simulink model "R7014E_Measure"  (R2025b)
settings: Solver=ode5  StartTime=0.0  StopTime=inf  RelTol=1e-3  EnableMultiTasking=on
undefined symbols (not defined in the file): Ad, Ao, At, Bd, Cd, g, h_0, h_1, h_1_V, h_2, h_2_V, National_Instruments, PCIe, Q, R, Ts
libraries: sldrtlib x2, simulink x2
settings Model: Creator=wolfgang  LastModifiedBy=Amar
settings Model: ModifiedHistory=|
  | Created an adjusted empty Simulink diagram for the lab assignments
  | in the course R0002E
settings SolverCC: AlgebraicLoopSolver=TrustRegion  AutoInsertRateTranBlk=on
settings DataIOCC: SaveFormat=Array  SignalLoggingSaveFormat=ModelDataLogs  SaveOutput=off  SignalLogging=off  DSMLogging=off  SaveTime=off  ReturnWorkspaceOutputs=off
settings OptimizationCC: ExpressionDepthLimit=2147483647.0  LifeSpan=inf
settings DebuggingCC: UnderspecifiedInitializationDetection=Classic  MergeDetectMultiDrivingBlocksExec=none  SolverPrmCheckMsg=warning  FcnCallInpInsideContextMsg=warning  UnconnectedInputMsg=warning  UnconnectedOutputMsg=warning  UnconnectedLineMsg=warning  StateNameClashWarn=warning  SFUnexpectedBacktrackingDiag=warning  SFNoUnconditionalDefaultTransitionDiag=warning  SFExecutionAtInitializationDiag=none  ArithmeticOperatorsInVariantConditions=warning
settings HardwareCC: ProdBitPerPointer=32.0  ProdBitPerSizeT=32.0  ProdBitPerPtrDiffT=32.0  ProdLargestAtomicFloat=None  ProdIntDivRoundTo=Undefined  ProdEndianess=Unspecified  ProdWordSize=32.0  ProdHWDeviceType=32-bit Generic
settings ModelReferenceCC: EnableRefExpFcnMdlSchedulingChecks=on  PropagateSignalLabelsOutOfModel=off
settings SFSimCC: SimUseLocalCustomCode=off  CustomCodeUndefinedFunction=UseInterfaceOnly
settings RTWCC: RTWUseLocalCustomCode=off  GPUComputeCapability=3.5
settings CodeAppCC: StateflowObjectComments=on
settings GRTTargetCC: TargetLangStandard=C89/C90 (ANSI)
settings ConfigComp: CovMetricSettings=dw  CovSaveCumulativeToWorkspaceVar=on  CovSaveSingleToWorkspaceVar=on  CovExternalEMLEnable=off  CovSFcnEnable=off

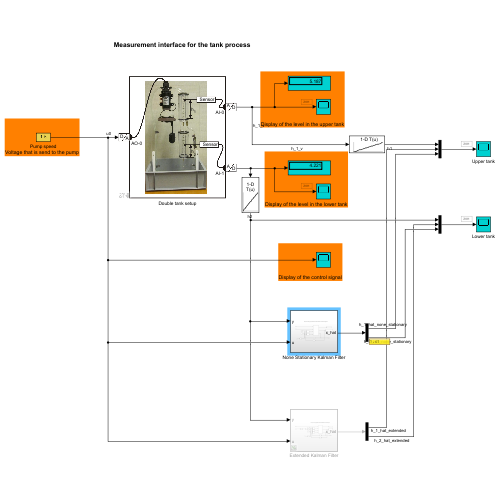
[thumbnail: Simulink's stored preview of the top-level diagram]
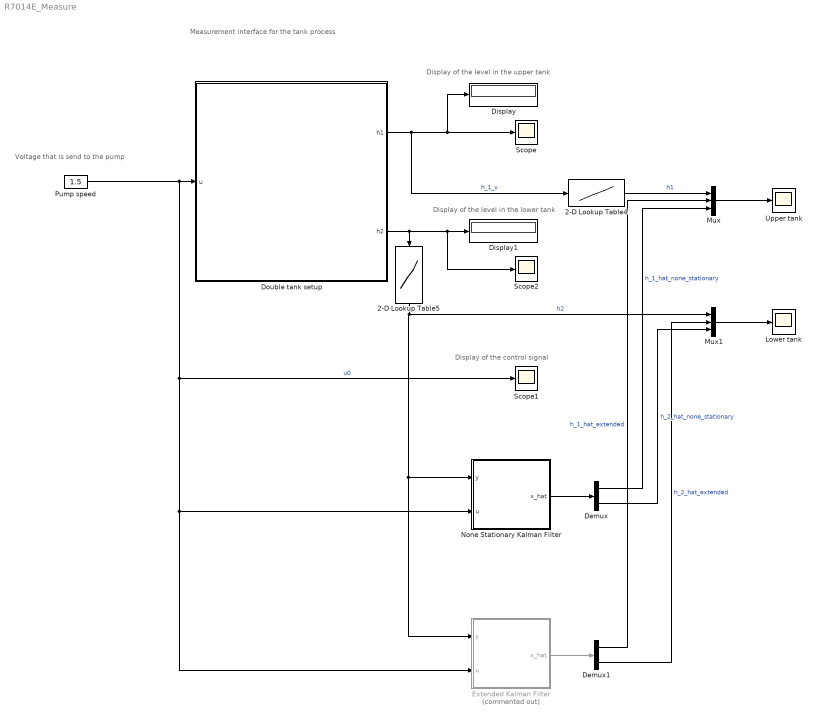
== system R7014E_Measure ==
  note: Measurement interface for the tank process
  note: Voltage that is send to the pump
  note: Display of the level in the upper tank
  note: Display of the control signal
  note: Display of the level in the lower tank
  2-D Lookup Table4 : Lookup_n-D  NumberOfTableDimensions=1  BreakpointsForDimension1=x  BreakpointsForDimension2=[1:3]  Table=y  RndMeth=Simplest  mask{x=h_1_V, y=h_1}
      mask prompts: x "Values on x-axis"; y "Values on y-axis"
  2-D Lookup Table5 : Lookup_n-D  NumberOfTableDimensions=1  BreakpointsForDimension1=x  BreakpointsForDimension2=[1:3]  Table=y  RndMeth=Simplest  mask{x=h_2_V, y=h_2}
      mask prompts: x "Values on x-axis"; y "Values on y-axis"
  Demux : Demux  Outputs=2
  Demux1 : Demux  Outputs=2
  Display : Display
  Display1 : Display
  Double tank setup : Subsystem  AncestorBlock=R0002E_lib/Double tank setup  mask(Realtime interface for the tank process){ts=Ts, h1_ch=0, h2_ch=1, u_ch=0}
      mask prompts: ts "Sample time"; h1_ch "A/D Channel for upper tank"; h2_ch "A/D Channel for lower tank"; u_ch "D/A Channel for pump"
      mask help:
      | This block represents the physical interface from the computer to the tank process.
      |
      | The input u is the voltage that is provided for the pump, the output h1 is the measured level in the upper tank in [V] and the output h2 is the
      | measured level in the lower tank in [V].
      |
      | You need to provide the sample rate at which the voltage to the pump is updated and the level measurements are sampled. The sample rate should not be less than 0.02 seconds.
      settings: LibrarySourceBlock=R0002E_lib/Double tank setup
      mask Display:
      | x=363;
      | y=381;
      | image(imread('tank_icon.jpg'));
      | text(250/x,309/y,'Sensor');
      | text(260/x,169/y,'Sensor');
      | text(335/x,289/y,'A');
      | text(351/x,283/y,'D');
      | text(335/x,100/y,'A');
      | text(351/x,95/y,'D');
      | text(22/x,187/y,'A');
      | text(5/x,195/y,'D');
      | text(225/x,278/y,'h_1','texmode','on');
      | text(225/x,146/y,'h_2','texmode','on');
      | text(300/x,270/y,sprintf('AI-%d',h1_ch));
      | text(300/x,80/y,sprintf('AI-%d',h2_ch));
      | text(40/x,173/y,sprintf('AO-%d',u_ch));
  Extended Kalman Filter : Subsystem  Commented=on
  Lower tank : Scope
      settings: SampleTime=0.1  TimeSpan=200  ActiveDisplayYMinimum=-4.8844046976277262  ActiveDisplayYMaximum=17.672626579116233  DataLoggingVariableName=ScopeData3  DataLoggingSaveFormat=Array
  Mux : Mux  Inputs=3
  Mux1 : Mux  Inputs=3
  None Stationary Kalman Filter : Subsystem
  Pump speed : Constant  Value=1.5
  Scope : Scope
      settings: SampleTime=0.1  TimeSpan=200  ActiveDisplayYMinimum=-1  ActiveDisplayYMaximum=1  DataLoggingSaveFormat=Array
  Scope1 : Scope
      settings: SampleTime=0.1  TimeSpan=200  ActiveDisplayYMinimum=0  DataLoggingSaveFormat=Array
  Scope2 : Scope
      settings: SampleTime=0.1  TimeSpan=200  ActiveDisplayYMinimum=0  ActiveDisplayYMaximum=20  DataLoggingVariableName=ScopeData2  DataLoggingSaveFormat=Array
  Upper tank : Scope
      settings: SampleTime=0.1  TimeSpan=200  ActiveDisplayYMinimum=-11.086400420135282  ActiveDisplayYMaximum=21.20768858424583  DataLoggingVariableName=ScopeData4  DataLoggingSaveFormat=Array
  wires:
  Pump speed/1 -> Extended Kalman Filter/2(u), None Stationary Kalman Filter/2(u), Scope1/1, Double tank setup/1(u)  "u0"
  Double tank setup/1(h1) -> 2-D Lookup Table4/1, Display/1, Scope/1  "h_1_v"
  Double tank setup/2(h2) -> 2-D Lookup Table5/1, Scope2/1, Display1/1
  None Stationary Kalman Filter/1(x_hat) -> Demux/1
  Demux/1 -> Mux/3  "h_1_hat_none_stationary"
  Demux/2 -> Mux1/3  "h_2_hat_none_stationary"
  Mux1/1 -> Lower tank/1
  Mux/1 -> Upper tank/1
  Extended Kalman Filter/1(x_hat) -> Demux1/1
  Demux1/1 -> Mux/2  "h_1_hat_extended"
  Demux1/2 -> Mux1/2  "h_2_hat_extended"
  2-D Lookup Table4/1 -> Mux/1  "h1"
  2-D Lookup Table5/1 -> Extended Kalman Filter/1(y), None Stationary Kalman Filter/1(y), Mux1/1  "h2"

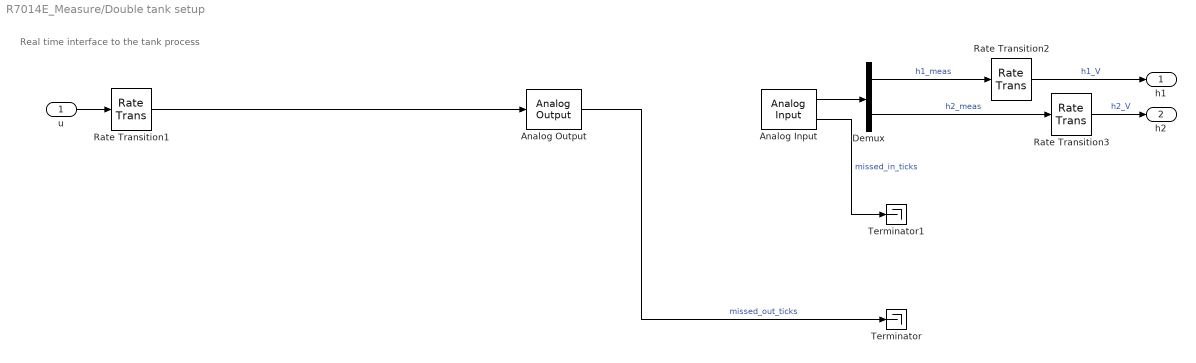
== system R7014E_Measure/Double tank setup ==
  note: Real time interface to the tank process
  u : Inport
  Analog Input : sldrtlib/Analog Input  SampleTime=ts  MaxMissedTicks=500000000  ShowMissedTicks=on  YieldWhenWaiting=off  DrvName=National_Instruments/PCIe-6321  DrvAddress=4294967295  DrvOptions=[0 0 0 0 0 0 0]  Channels=[h1_ch+1,h2_ch+1]  RangeMode=1  VoltRange=1  DataType=1
      settings: AttributesFormatString=National Instruments\nPCIe-6321 [auto]
  Analog Output : sldrtlib/Analog Output  SampleTime=ts  MaxMissedTicks=500000000  ShowMissedTicks=on  YieldWhenWaiting=off  DrvName=National_Instruments/PCIe-6321  DrvAddress=4294967295  DrvOptions=[0 0 0 0 0 0 0]  Channels=u_ch+1  RangeMode=1  VoltRange=1  InitialValue=0  FinalValue=0
      settings: AttributesFormatString=National Instruments\nPCIe-6321 [auto]
  Demux : Demux  Outputs=2
  Rate Transition1 : RateTransition  OutPortSampleTime=ts
  Rate Transition2 : RateTransition
  Rate Transition3 : RateTransition
  Terminator : Terminator
  Terminator1 : Terminator
  h1 : Outport
  h2 : Outport  Port=2
  wires:
  Rate Transition1/1 -> Analog Output/1
  Rate Transition3/1 -> h2/1  "h2_V"
  Rate Transition2/1 -> h1/1  "h1_V"
  Analog Input/2 -> Terminator1/1  "missed_in_ticks"
  Demux/2 -> Rate Transition3/1  "h2_meas"
  Demux/1 -> Rate Transition2/1  "h1_meas"
  Analog Input/1 -> Demux/1
  Analog Output/1 -> Terminator/1  "missed_out_ticks"
  u/1 -> Rate Transition1/1

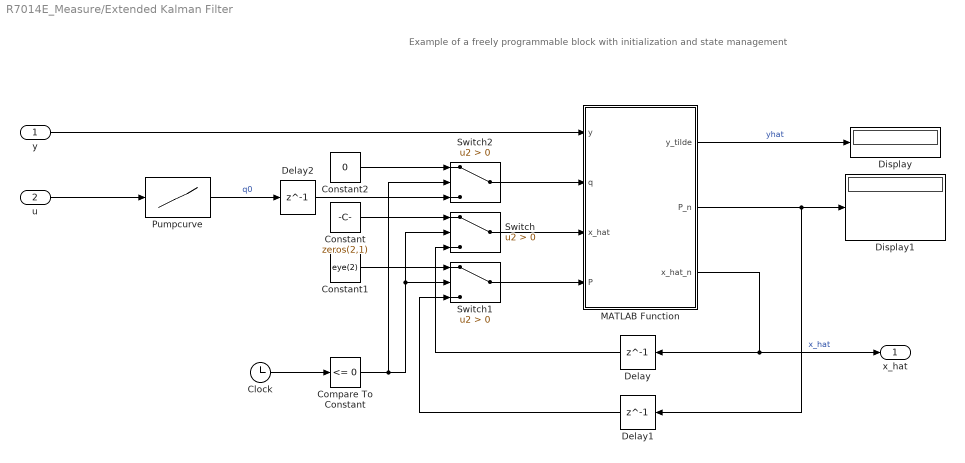
== system R7014E_Measure/Extended Kalman Filter ==
  note: Example of a freely programmable block with initialization and state management
  y : Inport
  u : Inport  Port=2
  Clock : Clock
  Compare To Constant : simulink/Logic and Bit Operations/Compare To Constant  relop=<=  const=0  OutDataTypeStr=boolean
  Constant : Constant  Value=zeros(2,1)
  Constant1 : Constant  Value=eye(2)
  Constant2 : Constant  Value=0
  Delay : Delay  DelayLength=1  InitialCondition=0
  Delay1 : Delay  DelayLength=1  InitialCondition=0
  Delay2 : Delay  DelayLength=1  InitialCondition=0
  Display : Display
  Display1 : Display
  MATLAB Function : MATLAB Function  TreatAsAtomicUnit=on
  Pumpcurve : Lookup_n-D  NumberOfTableDimensions=1  BreakpointsForDimension1=x  BreakpointsForDimension2=[1:3]  Table=y  RndMeth=Simplest  mask{x=[0.5,1,1.5,2,2.5,3,3.5,5,8,10], y=[16.47,20.75,24.52,27.63,30.06,32.49,34.80,40.28,48.24,52.43]}
      mask prompts: x "Values on x-axis"; y "Values on y-axis"
  Switch : Switch  Criteria=u2 > Threshold  SaturateOnIntegerOverflow=off  InputSameDT=off
  Switch1 : Switch  Criteria=u2 > Threshold  SaturateOnIntegerOverflow=off  InputSameDT=off
  Switch2 : Switch  Criteria=u2 > Threshold  SaturateOnIntegerOverflow=off  InputSameDT=off
  x_hat : Outport  PortDimensions=2
  wires:
  Delay/1 -> Switch/3
  Switch/1 -> MATLAB Function/3(x_hat)
  Constant1/1 -> Switch1/1
  Compare To Constant/1 -> Switch2/2, Switch/2, Switch1/2
  Constant/1 -> Switch/1
  MATLAB Function/1(y_tilde) -> Display/1  "yhat"
  MATLAB Function/2(P_n) -> Delay1/1, Display1/1
  Clock/1 -> Compare To Constant/1
  Switch1/1 -> MATLAB Function/4(P)
  y/1 -> MATLAB Function/1(y)
  Delay1/1 -> Switch1/3
  Switch2/1 -> MATLAB Function/2(q)
  Constant2/1 -> Switch2/1
  Delay2/1 -> Switch2/3
  Pumpcurve/1 -> Delay2/1  "q0"
  u/1 -> Pumpcurve/1
  MATLAB Function/3(x_hat_n) -> Delay/1, x_hat/1  "x_hat"

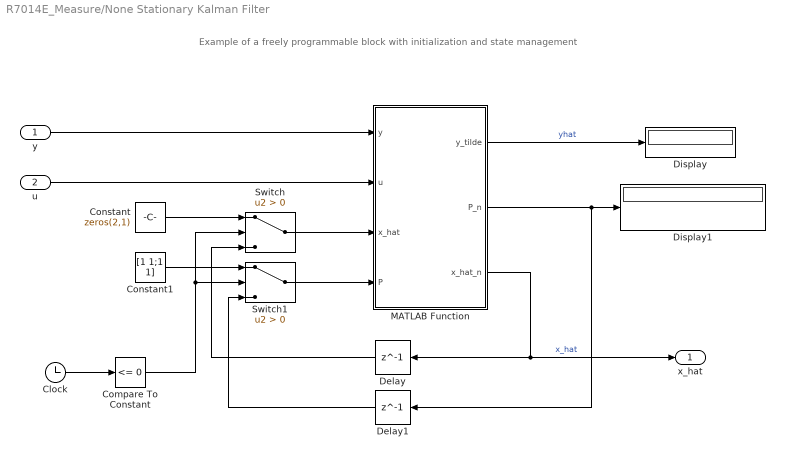
== system R7014E_Measure/None Stationary Kalman Filter ==
  note: Example of a freely programmable block with initialization and state management
  y : Inport
  u : Inport  Port=2
  Clock : Clock
  Compare To Constant : simulink/Logic and Bit Operations/Compare To Constant  relop=<=  const=0  OutDataTypeStr=boolean
  Constant : Constant  Value=zeros(2,1)
  Constant1 : Constant  Value=[1 1;1 1]
  Delay : Delay  DelayLength=1  InitialCondition=0
  Delay1 : Delay  DelayLength=1  InitialCondition=0
  Display : Display
  Display1 : Display
  MATLAB Function : MATLAB Function  TreatAsAtomicUnit=on
  Switch : Switch  Criteria=u2 > Threshold  SaturateOnIntegerOverflow=off  InputSameDT=off
  Switch1 : Switch  Criteria=u2 > Threshold  SaturateOnIntegerOverflow=off  InputSameDT=off
  x_hat : Outport  PortDimensions=2
  wires:
  Delay/1 -> Switch/3
  Switch/1 -> MATLAB Function/3(x_hat)
  Constant1/1 -> Switch1/1
  Compare To Constant/1 -> Switch1/2, Switch/2
  MATLAB Function/3(x_hat_n) -> x_hat/1, Delay/1  "x_hat"
  Constant/1 -> Switch/1
  MATLAB Function/1(y_tilde) -> Display/1  "yhat"
  MATLAB Function/2(P_n) -> Display1/1, Delay1/1
  Clock/1 -> Compare To Constant/1
  Switch1/1 -> MATLAB Function/4(P)
  y/1 -> MATLAB Function/1(y)
  Delay1/1 -> Switch1/3
  u/1 -> MATLAB Function/2(u)

== matlab function R7014E_Measure/None Stationary Kalman Filter/MATLAB Function ==
  data: y input; u input; x_hat input; y_tilde output; P input; P_n output; x_hat_n output; Ad parameter; Bd parameter; Cd parameter; Q parameter; R parameter
function [y_tilde, P_n, x_hat_n] = fcn(y, u, x_hat, P, Ad, Bd, Cd, Q, R)

% Predict
x_hat_n = Ad*x_hat + Bd*u;
P_n = Ad*P*Ad' + Q;

% Update
y_tilde = y - Cd*x_hat_n;
S = Cd*P_n*Cd' + R;
K = P_n*Cd'*inv(S);
x_hat_n = x_hat_n + K*y_tilde;
%P_n = (eye(2) - K*Cd)*P_n*(eye(2) - K*Cd)' + K*R*K'; %Joseph Form
P_n = (eye(2) - K*Cd)*P_n
y_tilde = y - Cd*x_hat_n;

== matlab function R7014E_Measure/Extended Kalman Filter/MATLAB Function ==
  data: y input; q input; x_hat input; y_tilde output; P input; P_n output; x_hat_n output; Q parameter; R parameter; Ao parameter; g parameter; At parameter; h_0 parameter; Ts parameter
function [y_tilde, P_n, x_hat_n] = fcn(y, q, x_hat, P, Q, R, Ao, g, At, h_0, Ts)

%Linearization
A = [-Ao*g*(1/(At*sqrt(2*g*(x_hat(1)+h_0)))) 0 ; 
    Ao*g*(1/(At*sqrt(2*g*(x_hat(1)+h_0)))) Ao*g*(-1/(At*sqrt(2*g*(x_hat(2)+h_0))))];
C = [0 1];

Ad = eye(size(A)) + Ts*A;
Cd = C;

% Predict
x_hat_dot = [q/At - Ao/At * sqrt(2*g*(x_hat(1) + h_0)); 
             Ao/At * sqrt(2*g*(x_hat(1) + h_0)) - Ao/At * sqrt(2*g*(x_hat(2) + h_0))];
x_hat_n = x_hat + x_hat_dot.*Ts;
P_n = Ad*P*Ad' + Q;


% Update
y_tilde = y - Cd*x_hat;
S = Cd*P_n*Cd' + R;
K = P_n*Cd'*inv(S);
x_hat_n = x_hat_n + K*y_tilde;
%P_n = (eye(2) - K*Cd)*P_n*(eye(2) - K*Cd)' + K*R*K'; %Joseph Form
P_n = (eye(2) - K*Cd)*P_n;   
y_tilde = y - Cd*x_hat_n;
